simulink model "Noble_Model_Complete"  (Simulink 8.1)
settings: Solver=ode45  StartTime=0.0  StopTime=5  RelTol=1e-3
libraries: simulink x1, simulink_extras x1
settings Model: Creator=Zack Tzeng  LastModifiedBy=User1
settings DataIOCC: SignalLoggingSaveFormat=Dataset
settings OptimizationCC: ExpressionDepthLimit=128
settings DebuggingCC: FcnCallInpInsideContextMsg=EnableAllAsError
settings GRTTargetCC: CombineOutputUpdateFcns=on  GRTInterface=off

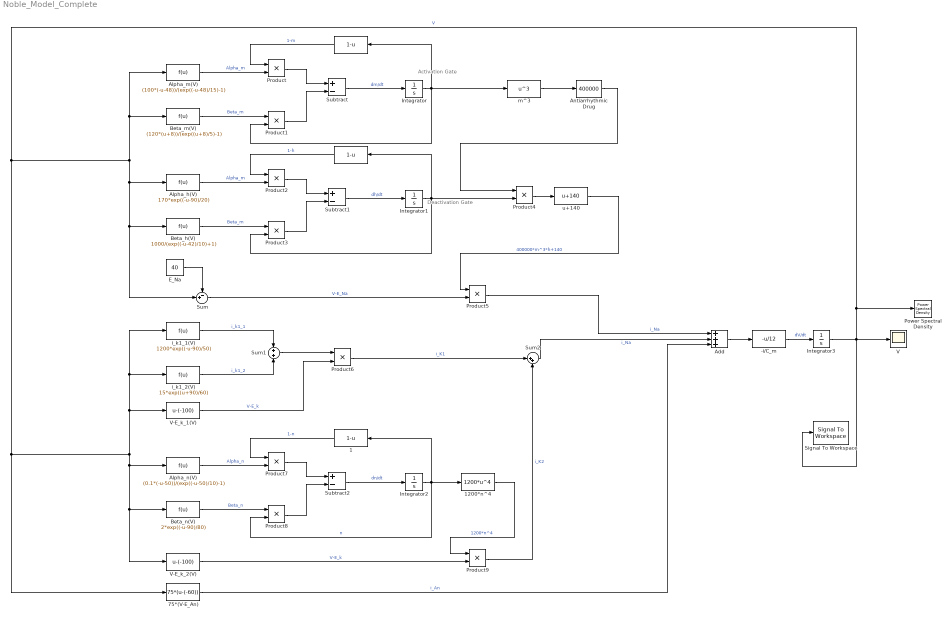
== system Noble_Model_Complete ==
  note: Deactivation
      | Gate
  note: Activation
      |     Gate
  " " : Fcn  Expr=1-u
  "  " : Fcn  Expr=1-u
  "  1" : Fcn  Expr=1-u
  -i/C_m : Fcn  Expr=-u/12
  "1200*n^4 " : Fcn  Expr=1200*u^4
  75*(V-E_An) : Fcn  Expr=75*(u-(-60))
  Add : Sum  Inputs=+++
  Alpha_h(V) : Fcn  Expr=170*exp((-u-90)/20)
  Alpha_m(V) : Fcn  Expr=(100*(-u-48))/(exp((-u-48)/15)-1)
  Alpha_n(V) : Fcn  Expr=(0.1*(-u-50))/(exp((-u-50)/10)-1)
  Antiarrhythmic Drug : simulink/Math Operations/Slider Gain  low=340000  gain=400000  high=400000
  Beta_h(V) : Fcn  Expr=1000/(exp((-u-42)/10)+1)
  Beta_m(V) : Fcn  Expr=(120*(u+8))/(exp((u+8)/5)-1)
  Beta_n(V) : Fcn  Expr=2*exp((-u-90)/80)
  E_Na : Constant  Value=40
  Integrator : Integrator  InitialCondition=0.04338  UpperSaturationLimit=500  LowerSaturationLimit=-500
  Integrator1 : Integrator  InitialCondition=0.85218  UpperSaturationLimit=500  LowerSaturationLimit=-500
  Integrator2 : Integrator  InitialCondition=0.60888  UpperSaturationLimit=500  LowerSaturationLimit=-500
  Integrator3 : Integrator  InitialCondition=-81.6  UpperSaturationLimit=500  LowerSaturationLimit=-500
  Power Spectral Density : simulink_extras/Additional Sinks/Power Spectral Density  npts=128  fftpts=512  HowOften=64  sampleT=0.1
  Product{,1..9} (10 alike) : Product
  Signal To Workspace : SignalToWorkspace  VariableName=Vout400000
      settings: CopyFcn=dspblkcopystw(gcbh);
  Subtract : Sum  Inputs=+-
  Subtract1 : Sum  Inputs=+-
  Subtract2 : Sum  Inputs=+-
  Sum : Sum  Inputs=-+|
  Sum1 : Sum  Inputs=+|+
  Sum2 : Sum  Inputs=|++
  V : Scope
  V-E_k_1(V) : Fcn  Expr=u-(-100)
  V-E_k_2(V) : Fcn  Expr=u-(-100)
  i_k1_1(V) : Fcn  Expr=1200*exp((-u-90)/50)
  i_k1_2(V) : Fcn  Expr=15*exp((u+90)/60)
  m^3 : Fcn  Expr=u^3
  "u+140 " : Fcn  Expr=u+140
  wires:
  E_Na/1 -> Sum/1
  Sum/1 -> Product5/2  "V-E_Na"
  Alpha_m(V)/1 -> Product/2  "Alpha_m"
  Beta_m(V)/1 -> Product1/1  "Beta_m"
  Integrator/1 -> m^3/1, " "/1, Product1/2
  Subtract/1 -> Integrator/1  "dm/dt"
  Product/1 -> Subtract/1
  Product1/1 -> Subtract/2
  Alpha_h(V)/1 -> Product2/2  "Alpha_m"
  Beta_h(V)/1 -> Product3/1  "Beta_m"
  Integrator1/1 -> "  "/1, Product4/2, Product3/2
  Subtract1/1 -> Integrator1/1  "dh/dt"
  Product2/1 -> Subtract1/1
  Product3/1 -> Subtract1/2
  " "/1 -> Product/1  "1-m"
  "  "/1 -> Product2/1  "1-h"
  Product4/1 -> "u+140 "/1
  m^3/1 -> Antiarrhythmic Drug/1
  "u+140 "/1 -> Product5/1  "400000*m^3*h+140"
  Product5/1 -> Add/1  "i_Na"
  V-E_k_2(V)/1 -> Product9/2  "V-E_k"
  i_k1_1(V)/1 -> Sum1/1  "i_k1_1"
  i_k1_2(V)/1 -> Sum1/2  "i_k1_2"
  Alpha_n(V)/1 -> Product7/2  "Alpha_n"
  Beta_n(V)/1 -> Product8/1  "Beta_n"
  Integrator2/1 -> "1200*n^4 "/1, "  1"/1, Product8/2  "n"
  Subtract2/1 -> Integrator2/1  "dn/dt"
  Product7/1 -> Subtract2/1
  Product8/1 -> Subtract2/2
  "  1"/1 -> Product7/1  "1-n"
  "1200*n^4 "/1 -> Product9/1  "1200*n^4"
  Product9/1 -> Sum2/2  "i_K2"
  Sum1/1 -> Product6/1
  V-E_k_1(V)/1 -> Product6/2  "V-E_k"
  Product6/1 -> Sum2/1  "i_K1"
  Sum2/1 -> Add/2  "i_Na"
  75*(V-E_An)/1 -> Add/3  "i_An"
  Add/1 -> -i/C_m/1
  -i/C_m/1 -> Integrator3/1  "dV/dt"
  Integrator3/1 -> Signal To Workspace/1, Power Spectral Density/1, V-E_k_2(V)/1, Beta_n(V)/1, Alpha_n(V)/1, V-E_k_1(V)/1, i_k1_2(V)/1, i_k1_1(V)/1, 75*(V-E_An)/1, Sum/2, Beta_h(V)/1, Alpha_h(V)/1, Beta_m(V)/1, Alpha_m(V)/1, V/1  "V"
  Antiarrhythmic Drug/1 -> Product4/1
